simulink model "PID_control_model"  (R2023b)
settings: Solver=VariableStepAuto  StartTime=0.0  StopTime=10.0  RelTol=1e-3
InitFcn:
  | B = 0.028;
  | K = 0.05;
  | L = 0.1;
  | R = 0.25;
  | J =  3.37e-5;
settings Model: Creator=Harish  LastModifiedBy=Harish

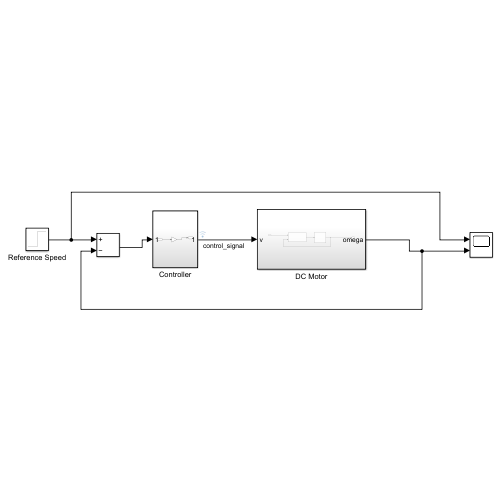
[thumbnail: Simulink's stored preview of the top-level diagram]
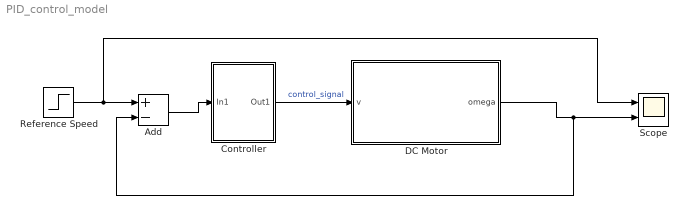
== system PID_control_model ==
  Add : Sum  Inputs=+-
  Controller : Subsystem
  DC Motor : Subsystem
  Reference Speed : Step  SampleTime=0
  Scope : Scope  NumInputPorts=2
  wires:
  DC Motor/1(omega) -> Add/2, Scope/2
  Add/1 -> Controller/1(In1)
  Controller/1(Out1) -> DC Motor/1(v)  "control_signal"
  Reference Speed/1 -> Scope/1, Add/1

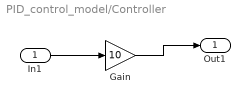
== system PID_control_model/Controller ==
  In1 : Inport
  Gain : Gain  Gain=10
  Out1 : Outport
  wires:
  Gain/1 -> Out1/1
  In1/1 -> Gain/1

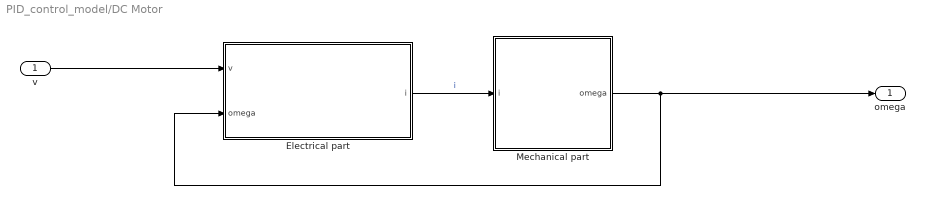
== system PID_control_model/DC Motor ==
  v : Inport
  "Electrical part " : Subsystem
  Mechanical part : Subsystem
  omega : Outport
  wires:
  "Electrical part "/1(i) -> Mechanical part/1(i)  "i"
  Mechanical part/1(omega) -> omega/1, "Electrical part "/2(omega)
  v/1 -> "Electrical part "/1(v)

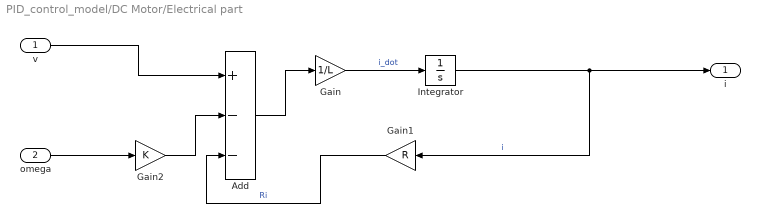
== system PID_control_model/DC Motor/Electrical part  ==
  v : Inport
  omega : Inport  Port=2
  Add : Sum  Inputs=+--
  Gain : Gain  Gain=1/L
  Gain1 : Gain  Gain=R
  Gain2 : Gain  Gain=K
  Integrator : Integrator
  i : Outport
  wires:
  Add/1 -> Gain/1
  Integrator/1 -> i/1, Gain1/1  "i"
  Gain1/1 -> Add/3  "Ri"
  v/1 -> Add/1
  Gain2/1 -> Add/2
  Gain/1 -> Integrator/1  "i_dot"
  omega/1 -> Gain2/1

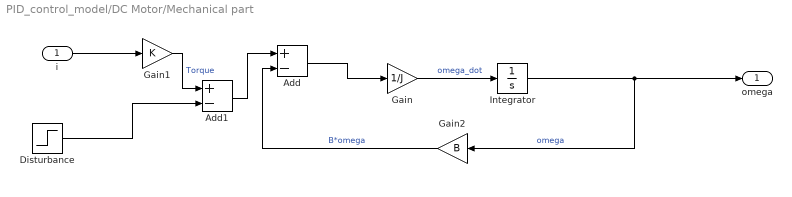
== system PID_control_model/DC Motor/Mechanical part ==
  i : Inport
  Add : Sum  Inputs=+-
  Add1 : Sum  Inputs=+-
  Disturbance : Step  Time=2  After=0.1  SampleTime=0
  Gain : Gain  Gain=1/J
  Gain1 : Gain  Gain=K
  Gain2 : Gain  Gain=B
  Integrator : Integrator
  omega : Outport
  wires:
  Add/1 -> Gain/1
  Integrator/1 -> omega/1, Gain2/1  "omega"
  Gain2/1 -> Add/2  "B*omega"
  i/1 -> Gain1/1
  Gain/1 -> Integrator/1  "omega_dot"
  Gain1/1 -> Add1/1  "Torque"
  Disturbance/1 -> Add1/2
  Add1/1 -> Add/1
